simulink model "gravcomp"  (Simulink 7.5)
settings: Solver=ode3  StartTime=0.0  StopTime=inf  FixedStep=.002  RelTol=1e-3
undefined symbols (not defined in the file or in its folder): arm_home, arm_j2mt, arm_m2jp, bit, CAN_init, enc_per_rev, fdesignblkfcn, FT_init, gcbh, hand_on, MT_init, puck_I_per_Nm, rotFT2Hand, sample_time, Standard, VL1_init, VL2_init
libraries: simulink x358, xpclib x28, xpcutilitieslib x6, dspmathops x1
(part 1 of 3)
settings Model: Creator=Matt Courtney  LastModifiedBy=robotics  BufferReuse=off
settings OptimizationCC: BlockReduction=off  BooleanDataType=off  OptimizeBlockIOStorage=off  BufferReuse=off  ExpressionFolding=off  LocalBlockOutputs=off  InitFltsAndDblsToZero=on
settings DebuggingCC: StrictBusMsg=Warning
settings HardwareCC: ProdIntDivRoundTo=Zero  ProdEndianess=LittleEndian  ProdHWDeviceType=Generic->32-bit x86 compatible
settings RTWCC: SystemTargetFile=xpctarget.tlc  TemplateMakefile=xpc_default_tmf  Description=xPC Target  ProcessScript=xpctarget_make_rtw_hook  RTWCompilerOptimization=On
settings xpcTargetCC: TargetFcnLib=ansi_tfl_table_tmw.mat  TargetFunctionLibrary=ANSI_C  ERTCodeCoverageTool=None  ParMdlRefBuildCompliant=off  PortableWordSizes=off  xPCisModelTimeout=off  xPCModelTimeoutSecs=10  xPCLoadParamSetFile=off

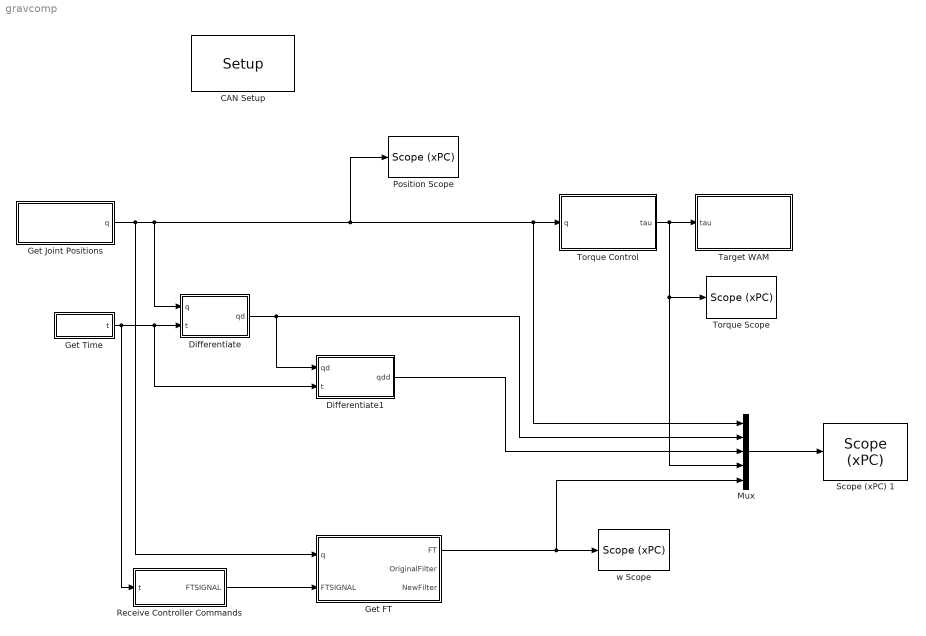
== system gravcomp ==
  "CAN Setup " : xpclib/CAN/Softing/CAN-AC2-PCI SJA 1000/Setup   board=1  can1bus=Highspeed (ISO 11898)  can1Baudrate=1 MBaud  can1UserBR=[1,1,4,3]  can2bus=Highspeed (ISO 11898)  can2Baudrate=1 MBaud  can2UserBR=[1,1,4,3]  init=[VL1_init,VL2_init,CAN_init,FT_init,MT_init]  term=[]  bus_off_out=off  bus_off_rec=Off  ioBaseAddress=-1
  Differentiate : Subsystem
  Differentiate1 : Subsystem
  Get FT : Subsystem
  Get Joint Positions : Subsystem
  Get Time : Subsystem
  Mux : Mux  Inputs=[7 7 7 7 6]
  Position Scope : xpclib/Misc./Scope (xPC)   SystemSampleTime=-1  scopeno=5  scopetype=Target  autostart=on  viewmode=Numerical  formatstr=['joint_1 %13.8f rad,joint_2 %13.8f rad,joint_3 %13.8f rad,joint_4 %13.8f rad,joint_5 %13.8f rad,joint_6 %13.8f rad,joint_7 %13.8f rad']  grid=on  ylimits=[0,0]  nosamples=1/(10*sample_time)  noprepostsamples=0  interleave=1  triggermode=FreeRun  triggersignal=1  triggerlevel=0.0  triggerslope=Either  triggerscope=1  triggersample=0  filename=data.dat  mode=Lazy  writesize=512  autorestart=off  dynamicfilemode=off  maxwritefilesize=512*1024^2
  Receive Controller Commands : Subsystem
  Scope (xPC) 1 : xpclib/Misc./Scope (xPC)   SystemSampleTime=-1  scopeno=6  scopetype=File  autostart=on  viewmode=Graphical redraw  formatstr='%15.6f'  grid=on  ylimits=[0,0]  nosamples=250  noprepostsamples=0  interleave=1  triggermode=FreeRun  triggersignal=1  triggerlevel=0.0  triggerslope=Either  triggerscope=1  triggersample=0  filename=GRAV<%%%>.dat  mode=Lazy  writesize=512  autorestart=on  dynamicfilemode=on  maxwritefilesize=512*1024^2
  Target WAM : Subsystem
  Torque Control : Subsystem
  Torque Scope : xpclib/Misc./Scope (xPC)   SystemSampleTime=-1  scopeno=1  scopetype=Target  autostart=on  viewmode=Numerical  formatstr=['joint_1 %10.5f N-m,joint_2 %10.5f N-m,joint_3 %10.5f N-m,joint_4 %10.5f N-m,joint_5 %10.5f N-m,joint_6 %10.5f N-m,joint_7 %10.5f N-m']  grid=on  ylimits=[0,0]  nosamples=1/(10*sample_time)  noprepostsamples=0  interleave=1  triggermode=FreeRun  triggersignal=1  triggerlevel=0.0  triggerslope=Either  triggerscope=1  triggersample=0  filename=data.dat  mode=Lazy  writesize=512  autorestart=off  dynamicfilemode=off  maxwritefilesize=512*1024^2
  w Scope : xpclib/Misc./Scope (xPC)   SystemSampleTime=-1  scopeno=2  scopetype=Target  autostart=on  viewmode=Numerical  formatstr=['Fx %10.5f,Fy %10.5f,Fz %10.5f,TauX %10.5f,TauY %10.5f,TauZ%10.5f']  grid=on  ylimits=[0,0]  nosamples=10  noprepostsamples=0  interleave=1  triggermode=FreeRun  triggersignal=1  triggerlevel=0.0  triggerslope=Either  triggerscope=1  triggersample=0  filename=data.dat  mode=Lazy  writesize=512  autorestart=off  dynamicfilemode=off  maxwritefilesize=512*1024^2
  wires:
  Torque Control/1(tau) -> Target WAM/1(tau), Mux/4, Torque Scope/1
  Get Joint Positions/1(q) -> Differentiate/1(q), Torque Control/1(q), Mux/1, Position Scope/1, Get FT/1(q)
  Get FT/1(FT) -> w Scope/1, Mux/5
  Mux/1 -> Scope (xPC) 1/1
  Get Time/1(t) -> Differentiate/2(t), Differentiate1/2(t), Receive Controller Commands/1(t)
  Differentiate/1(qd) -> Differentiate1/1(qd), Mux/2
  Differentiate1/1(qdd) -> Mux/3
  Receive Controller Commands/1(FTSIGNAL) -> Get FT/2(FTSIGNAL)

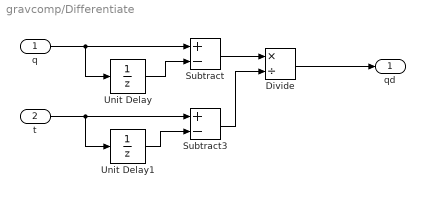
== system gravcomp/Differentiate ==
  q : Inport  OutDataType=fixdt(1, 16)  OutScaling=2^0
  t : Inport  Port=2  OutDataType=fixdt(1, 16)  OutScaling=2^0
  Divide : Product  Inputs=*/  OutDataType=fixdt(1, 16)  OutScaling=2^-10
  Subtract : Sum  Inputs=+-  OutDataType=fixdt(1, 16)  OutScaling=2^-10
  Subtract3 : Sum  Inputs=+-  OutDataType=fixdt(1, 16)  OutScaling=2^-10
  Unit Delay : UnitDelay  SampleTime=-1
  Unit Delay1 : UnitDelay  SampleTime=-1
  qd : Outport  OutDataType=fixdt(1, 16)  OutScaling=2^0
  wires:
  q/1 -> Subtract/1, Unit Delay/1
  t/1 -> Unit Delay1/1, Subtract3/1
  Unit Delay1/1 -> Subtract3/2
  Unit Delay/1 -> Subtract/2
  Subtract/1 -> Divide/1
  Divide/1 -> qd/1
  Subtract3/1 -> Divide/2

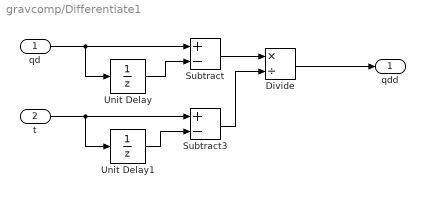
== system gravcomp/Differentiate1 ==
  qd : Inport  OutDataType=fixdt(1, 16)  OutScaling=2^0
  t : Inport  Port=2  OutDataType=fixdt(1, 16)  OutScaling=2^0
  Divide : Product  Inputs=*/  OutDataType=fixdt(1, 16)  OutScaling=2^-10
  Subtract : Sum  Inputs=+-  OutDataType=fixdt(1, 16)  OutScaling=2^-10
  Subtract3 : Sum  Inputs=+-  OutDataType=fixdt(1, 16)  OutScaling=2^-10
  Unit Delay : UnitDelay  SampleTime=-1
  Unit Delay1 : UnitDelay  SampleTime=-1
  qdd : Outport  OutDataType=fixdt(1, 16)  OutScaling=2^0
  wires:
  qd/1 -> Subtract/1, Unit Delay/1
  t/1 -> Unit Delay1/1, Subtract3/1
  Unit Delay1/1 -> Subtract3/2
  Unit Delay/1 -> Subtract/2
  Subtract/1 -> Divide/1
  Divide/1 -> qdd/1
  Subtract3/1 -> Divide/2

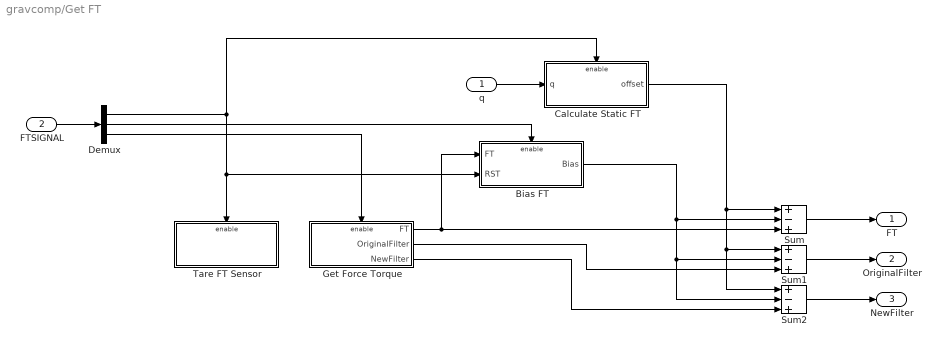
== system gravcomp/Get FT ==
  q : Inport  OutDataType=fixdt(1, 16)  OutScaling=2^0
  FTSIGNAL : Inport  Port=2  OutDataType=fixdt(1, 16)  OutScaling=2^0
  Bias FT : Subsystem  TreatAsAtomicUnit=on
  Calculate Static FT : Subsystem  TreatAsAtomicUnit=on
  Demux : Demux  Outputs=3
  Get Force Torque : Subsystem
  Sum : Sum  Inputs=+-+  OutDataType=fixdt(1, 16)  OutScaling=2^0
  Sum1 : Sum  Inputs=+-+  OutDataType=fixdt(1, 16)  OutScaling=2^0
  Sum2 : Sum  Inputs=+-+  OutDataType=fixdt(1, 16)  OutScaling=2^0
  Tare FT Sensor : Subsystem  TreatAsAtomicUnit=on
  FT : Outport  OutDataType=fixdt(1, 16)  OutScaling=2^0
  OriginalFilter : Outport  Port=2  OutDataType=fixdt(1, 16)  OutScaling=2^0
  NewFilter : Outport  Port=3  OutDataType=fixdt(1, 16)  OutScaling=2^0
  wires:
  FTSIGNAL/1 -> Demux/1
  Demux/1 -> Tare FT Sensor/Enable, Bias FT/2(RST), Calculate Static FT/Enable
  Demux/3 -> Get Force Torque/Enable
  Demux/2 -> Bias FT/Enable
  Get Force Torque/1(FT) -> Bias FT/1(FT), Sum/3
  Sum/1 -> FT/1
  Bias FT/1(Bias) -> Sum/2, Sum2/2, Sum1/2
  Get Force Torque/2(OriginalFilter) -> Sum1/3
  Get Force Torque/3(NewFilter) -> Sum2/3
  Sum2/1 -> NewFilter/1
  Sum1/1 -> OriginalFilter/1
  q/1 -> Calculate Static FT/1(q)
  Calculate Static FT/1(offset) -> Sum/1, Sum1/1, Sum2/1

== system gravcomp/Get Joint Positions ==
  DocBlock : simulink/Model-Wide Utilities/DocBlock  SystemSampleTime=-1  DocumentType=Text
  Motor Counts to Joint Radians1 : Subsystem
  Recieve and Unpack  Motor Positions1 : Subsystem
  Send: GetPosition : Subsystem
  q : Outport  OutDataType=sfix(16)  OutScaling=2^0
  wires:
  Motor Counts to Joint Radians1/1(qJ) -> q/1
  Recieve and Unpack  Motor Positions1/1(qM) -> Motor Counts to Joint Radians1/1(qM)

== system gravcomp/Get Time ==
  Clock Frequency : Constant  Value=1.193e6  OutDataType=fixdt(1, 16)  OutScaling=2^0
  Divide1 : Product  Inputs=*/  OutDataType=fixdt(1, 16)  OutScaling=2^-10
  "xPC Target  Time " : xpclib/Misc./xPC Target  Time   ts=sample_time
  t : Outport  OutDataType=fixdt(1, 16)  OutScaling=2^0
  wires:
  "xPC Target  Time "/1 -> Divide1/1
  Clock Frequency/1 -> Divide1/2
  Divide1/1 -> t/1

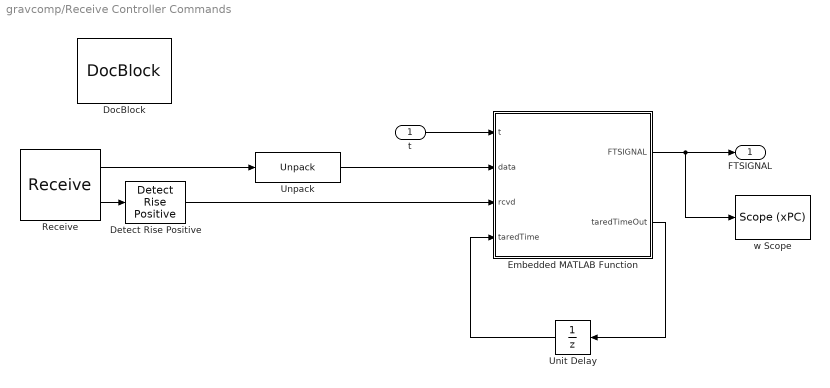
== system gravcomp/Receive Controller Commands ==
  t : Inport  OutDataType=fixdt(1, 16)  OutScaling=2^0
  Detect Rise Positive : simulink/Logic and Bit Operations/Detect Rise Positive  SystemSampleTime=-1  vinit=0
  DocBlock : simulink/Model-Wide Utilities/DocBlock  SystemSampleTime=-1  DocumentType=Text
  Embedded MATLAB Function : Stateflow chart  TreatAsAtomicUnit=on
  Receive : xpclib/UDP/Receive  ipAddress=192.168.1.11  ipPort=6666  width=9  vblLen=off  sampletime=sample_time
  Unit Delay : UnitDelay  SampleTime=-1
  Unpack : xpclib/UDP/Unpack  dimensions={[9,1]}  datatypes={'uint8'}  byteAlign=1
  w Scope : xpclib/Misc./Scope (xPC)   SystemSampleTime=-1  scopeno=3  scopetype=Target  autostart=on  viewmode=Numerical  formatstr=['%10.5f']  grid=on  ylimits=[0,0]  nosamples=10  noprepostsamples=0  interleave=1  triggermode=FreeRun  triggersignal=1  triggerlevel=0.0  triggerslope=Either  triggerscope=1  triggersample=0  filename=data.dat  mode=Lazy  writesize=512  autorestart=off  dynamicfilemode=off  maxwritefilesize=512*1024^2
  FTSIGNAL : Outport  OutDataType=fixdt(1, 16)  OutScaling=2^0
  wires:
  Receive/1 -> Unpack/1
  Receive/2 -> Detect Rise Positive/1
  Detect Rise Positive/1 -> Embedded MATLAB Function/3(rcvd)
  Unpack/1 -> Embedded MATLAB Function/2(data)
  t/1 -> Embedded MATLAB Function/1(t)
  Embedded MATLAB Function/2(taredTimeOut) -> Unit Delay/1
  Unit Delay/1 -> Embedded MATLAB Function/4(taredTime)
  Embedded MATLAB Function/1(FTSIGNAL) -> FTSIGNAL/1, w Scope/1

== system gravcomp/Target WAM ==
  tau : Inport  OutDataType=sfix(16)  OutScaling=2^0
  Check WAM MODE : Subsystem
  DocBlock : simulink/Model-Wide Utilities/DocBlock  SystemSampleTime=-1  DocumentType=Text
      content=|
      | This block does all of the communication with the WAM over the CAN card.
      | First we check the WAM mode to see if it in is Shift-Idle or Shift-Active
      | mode. It is necessary to pass this as output, so that PID knows whether it
      | should be integrating on the error or not. If we are in Shift-Idle mode,
      | we send zero torques. Also in this block, we convert joint torque to motor
      | current using the transformations in the documentation. Then we pack the
      | torque packets into a CAN message and send it.
      |
      | To receive joint positions we also send a CAN message which will respond
      | back with the appropriate information. Once we receive the joint positions,
      | we need to differentiate it to get joint velocities (since the WAM does not
      | have tachometers). Finally, passing it through a moving average of the last
      | n readings removes some of the noise and gives us a smoother velocity
      | signal.
  Joint Torque to Motor Current1 : Subsystem
  Pack and Send Torque Packets : Subsystem
  Switch : Switch  Threshold=2  OutDataType=sfix(16)  OutScaling=2^0
  Zero Torques : Constant  Value=[ 0 0 0 0 0 0 0]'  OutDataTypeMode=int16  OutDataType=sfix(16)  OutScaling=2^0  OutDataTypeStr=int16
  wires:
  Joint Torque to Motor Current1/1(iM) -> Pack and Send Torque Packets/1(Current)
  Switch/1 -> Joint Torque to Motor Current1/1(tauJ)
  tau/1 -> Switch/1
  Zero Torques/1 -> Switch/3
  Check WAM MODE/1(MODE) -> Switch/2

== system gravcomp/Torque Control ==
  q : Inport  OutDataType=sfix(16)  OutScaling=2^0
  Constant1 : Constant  Value=hand_on  OutDataType=fixdt(1, 16)  OutScaling=2^0
  Gravity Comp : Stateflow chart  TreatAsAtomicUnit=on
  tau : Outport  OutDataType=sfix(16)  OutScaling=2^0
  wires:
  q/1 -> Gravity Comp/2(q)
  Gravity Comp/1(tau) -> tau/1
  Constant1/1 -> Gravity Comp/1(hand_on)

== system gravcomp/Get FT/Bias FT ==
  FT : Inport  OutDataType=fixdt(1, 16)  OutScaling=2^0
  RST : Inport  Port=2  OutDataType=fixdt(1, 16)  OutScaling=2^0
  Enable : EnablePort  StatesWhenEnabling=reset
  Constant : Constant  Value=500  OutDataType=fixdt(1, 16)  OutScaling=2^0
  Cumulative Sum : dspmathops/Cumulative Sum  DialogController=dspDDGCreate  DialogControllerArgs=DataTag0  dim=Channels (running sum)  reset_popup=Non-zero sample  outputDataTypeStr=Inherit: Same as accumulator  outputLastDataTypeStr=Inherit: Same as accumulator  outputMin=[]  outputMax=[]  roundingMode=Floor  overflowMode=off
  Product : Product  Inputs=*/  OutDataType=fixdt(1, 16)  OutScaling=2^0  RndMeth=Zero
  Bias : Outport  OutDataType=fixdt(1, 16)  OutScaling=2^0
  wires:
  FT/1 -> Cumulative Sum/1
  RST/1 -> Cumulative Sum/2
  Constant/1 -> Product/2
  Cumulative Sum/1 -> Product/1
  Product/1 -> Bias/1

== system gravcomp/Get FT/Calculate Static FT ==
  q : Inport  OutDataType=fixdt(1, 16)  OutScaling=2^0
  Enable : EnablePort  StatesWhenEnabling=reset
  Constant1 : Constant  Value=hand_on  OutDataType=fixdt(1, 16)  OutScaling=2^0
  StaticFT : Stateflow chart  TreatAsAtomicUnit=on
  offset : Outport  OutDataType=fixdt(1, 16)  OutScaling=2^0
  wires:
  q/1 -> StaticFT/1(q)
  StaticFT/1(FTExp) -> offset/1
  Constant1/1 -> StaticFT/2(hand_on)

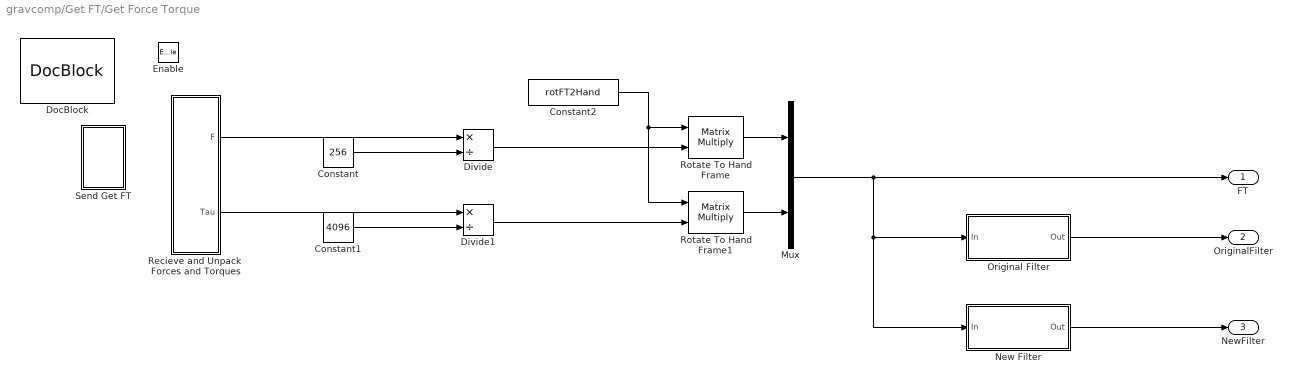
== system gravcomp/Get FT/Get Force Torque ==
  Enable : EnablePort
  Constant : Constant  Value=256  OutDataType=fixdt(1, 16)  OutScaling=2^0
  Constant1 : Constant  Value=4096  OutDataType=fixdt(1, 16)  OutScaling=2^0
  Constant2 : Constant  Value=rotFT2Hand  OutDataType=fixdt(1, 16)  OutScaling=2^0
  Divide : Product  Inputs=*/  OutDataType=fixdt(1, 16)  OutScaling=2^-10
  Divide1 : Product  Inputs=*/  OutDataType=fixdt(1, 16)  OutScaling=2^-10
  DocBlock : simulink/Model-Wide Utilities/DocBlock  SystemSampleTime=-1  DocumentType=Text
  Mux : Mux  Inputs=2
  New Filter : Subsystem  DialogController=fdesignblkfcn  DialogControllerArgs=DataTag3  InitFcn=fdesignblkfcn(gcbh, {'InitFcn'});
      settings: CopyFcn=fdesignblkfcn(gcbh, {'CopyFcn'});
      mask Type: Lowpass Filter
      mask Description: Design a lowpass filter
      mask Help: helpview(mapfilelocation('dspblks'), 'dsplowpassfilter')
      mask Display: disp('Lowpass')
  Original Filter : Subsystem  DialogController=fdesignblkfcn  DialogControllerArgs=DataTag6  InitFcn=fdesignblkfcn(gcbh, {'InitFcn'});
      settings: CopyFcn=fdesignblkfcn(gcbh, {'CopyFcn'});
      mask Type: Lowpass Filter
      mask Description: Design a lowpass filter
      mask Help: helpview(mapfilelocation('dspblks'), 'dsplowpassfilter')
      mask Display: disp('Lowpass')
  Recieve and Unpack  Forces and Torques : Subsystem
  Rotate To Hand Frame : Product  Multiplication=Matrix(*)  OutDataType=sfix(16)  OutScaling=2^0
  Rotate To Hand Frame1 : Product  Multiplication=Matrix(*)  OutDataType=sfix(16)  OutScaling=2^0
  Send Get FT : Subsystem
  FT : Outport  OutDataType=fixdt(1, 16)  OutScaling=2^0
  OriginalFilter : Outport  Port=2  OutDataType=fixdt(1, 16)  OutScaling=2^0
  NewFilter : Outport  Port=3  OutDataType=fixdt(1, 16)  OutScaling=2^0
  wires:
  Constant/1 -> Divide/2
  Constant1/1 -> Divide1/2
  Rotate To Hand Frame/1 -> Mux/1
  Rotate To Hand Frame1/1 -> Mux/2
  Constant2/1 -> Rotate To Hand Frame1/1, Rotate To Hand Frame/1
  Recieve and Unpack  Forces and Torques/2(Tau) -> Divide1/1
  Recieve and Unpack  Forces and Torques/1(F) -> Divide/1
  Divide/1 -> Rotate To Hand Frame/2
  Divide1/1 -> Rotate To Hand Frame1/2
  Mux/1 -> FT/1, New Filter/1(In), Original Filter/1(In)
  Original Filter/1(Out) -> OriginalFilter/1
  New Filter/1(Out) -> NewFilter/1

== system gravcomp/Get FT/Tare FT Sensor ==
  Enable : EnablePort
  ANY VALUE : Constant  Value=[0]  OutDataTypeMode=uint8  OutDataType=sfix(16)  OutScaling=2^0  OutDataTypeStr=uint8
  Bit Packing : xpcutilitieslib/Bit Packing   MaskBitPatterns={[0:7] [8:39] [40:55]}  MaskPackDataType=double  MaskPackDataSize=[1]
  Data Type Conversion1 : DataTypeConversion  OutMin=[-8191]  OutMax=[8191]  OutDataTypeMode=int32  OutDataType=int14  OutDataTypeStr=int32  RndMeth=Zero
  Send To FT : xpclib/CAN/Softing/CAN-AC2-PCI SJA 1000/Send   board=1  canPort=CAN 1  range=Standard (11-bit)  ids=bin2dec('00000001000')  sizes=[8]  output=off  ts=sample_time  ididx=[0]
  TARE FT : Constant  Value=[182]  OutDataTypeMode=uint8  OutDataType=sfix(16)  OutScaling=2^0  OutDataTypeStr=uint8
  wires:
  TARE FT/1 -> Bit Packing/1
  Bit Packing/1 -> Send To FT/1
  ANY VALUE/1 -> Data Type Conversion1/1
  Data Type Conversion1/1 -> Bit Packing/2, Bit Packing/3

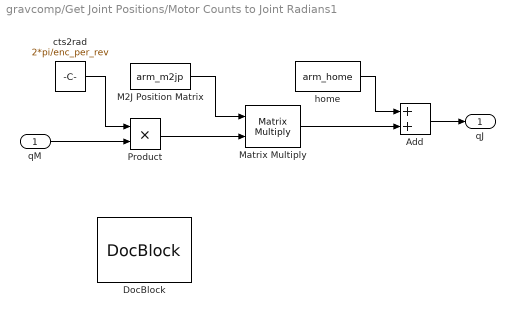
== system gravcomp/Get Joint Positions/Motor Counts to Joint Radians1 ==
  qM : Inport  OutDataType=fixdt(1, 16)  OutScaling=2^0
  Add : Sum  OutDataType=fixdt(1, 16)  OutScaling=2^-10
  DocBlock : simulink/Model-Wide Utilities/DocBlock  SystemSampleTime=-1  DocumentType=Text
      content=|
      | Here we do the simple conversion from motor position to joint position,
      | then convert encoder counts to joint radians, then account for the offset
      | in the home position to finally output the joint position in radians. The
      | M2J position matrix can be found in the documentation. Joint 4 has a -18 as
      | opposed to +18 because the motor was reversed at one point during a repair.
      | I believe newer models of the WAM adhere to this -18.
  M2J Position Matrix : Constant  Value=arm_m2jp  OutDataType=fixdt(1, 16)  OutScaling=2^0
  Matrix Multiply : Product  Multiplication=Matrix(*)  OutDataType=sfix(16)  OutScaling=2^0
  Product : Product  OutMin=[-8192]  OutMax=[8191]  OutDataType=fixdt(1, 16)  OutScaling=2^0  RndMeth=Zero
  cts2rad : Constant  Value=2*pi/enc_per_rev  OutDataType=fixdt(1, 16)  OutScaling=2^0
  home : Constant  Value=arm_home  OutDataType=fixdt(1, 16)  OutScaling=2^0
  qJ : Outport  OutDataType=fixdt(1, 16)  OutScaling=2^0
  wires:
  qM/1 -> Product/2
  Add/1 -> qJ/1
  Matrix Multiply/1 -> Add/2
  home/1 -> Add/1
  cts2rad/1 -> Product/1
  M2J Position Matrix/1 -> Matrix Multiply/1
  Product/1 -> Matrix Multiply/2

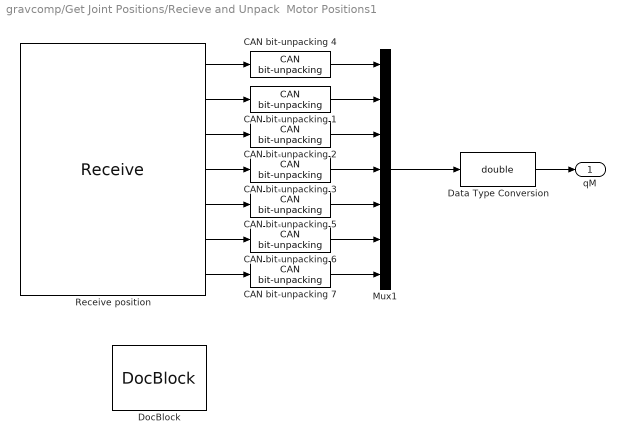
== system gravcomp/Get Joint Positions/Recieve and Unpack  Motor Positions1 ==
  CAN bit-unpacking {1..7} (7 alike) : xpclib/CAN/Utilities/CAN bit-unpacking   bitpatterns={ [16:23, 8:15, 0:5,-1, -1] }  dtypes={ 'int32'}
  Data Type Conversion : DataTypeConversion  OutDataTypeMode=double  OutDataType=sfix(16)  OutScaling=2^0  OutDataTypeStr=double
  DocBlock : simulink/Model-Wide Utilities/DocBlock  SystemSampleTime=-1  DocumentType=Text
  Mux1 : Mux  Inputs=7
  "Receive position " : xpclib/CAN/Softing/CAN-AC2-PCI SJA 1000/Receive   board=1  canPort=CAN 1  range=Standard (11-bit)  ids=[bin2dec('10000100011'),bin2dec('10001000011'),bin2dec('10001100011'),bin2dec('10010000011'),bin2dec('10010100011'),bin2dec('10011000011'),bin2dec('10011100011')]  lengths=0  output=Data  inten=on  ts=sample_time  ididx=[0,1,2,3,5,6,7]
  qM : Outport
  wires:
  Mux1/1 -> Data Type Conversion/1
  "Receive position "/1 -> CAN bit-unpacking 4/1
  "Receive position "/2 -> CAN bit-unpacking 1/1
  "Receive position "/3 -> CAN bit-unpacking 2/1
  "Receive position "/4 -> CAN bit-unpacking 3/1
  CAN bit-unpacking 4/1 -> Mux1/1
  CAN bit-unpacking 1/1 -> Mux1/2
  CAN bit-unpacking 2/1 -> Mux1/3
  CAN bit-unpacking 3/1 -> Mux1/4
  Data Type Conversion/1 -> qM/1
  "Receive position "/5 -> CAN bit-unpacking 5/1
  "Receive position "/6 -> CAN bit-unpacking 6/1
  "Receive position "/7 -> CAN bit-unpacking 7/1
  CAN bit-unpacking 5/1 -> Mux1/5
  CAN bit-unpacking 6/1 -> Mux1/6
  CAN bit-unpacking 7/1 -> Mux1/7

== system gravcomp/Get Joint Positions/Send: GetPosition ==
  Bit Packing : xpcutilitieslib/Bit Packing   MaskBitPatterns={[0:7]}  MaskPackDataType=double  MaskPackDataSize=[1]
  DocBlock : simulink/Model-Wide Utilities/DocBlock  SystemSampleTime=-1  DocumentType=Text
  Send to all motors : xpclib/CAN/Softing/CAN-AC2-PCI SJA 1000/Send   board=1  canPort=CAN 1  range=Standard (11-bit)  ids=1024  sizes=[1]  output=off  ts=sample_time  ididx=[2]
  get position : Constant  Value=[48]  OutDataTypeMode=int8  OutDataType=sfix(16)  OutScaling=2^0  OutDataTypeStr=int8
  wires:
  Bit Packing/1 -> Send to all motors/1
  get position/1 -> Bit Packing/1

== system gravcomp/Target WAM/Check WAM MODE ==
  note: Send to lower arm
  "Bit Packing " : xpcutilitieslib/Bit Packing   MaskBitPatterns={[0:7]}  MaskPackDataType=double  MaskPackDataSize=[1]
  Bit Unpacking : xpclib/CAN/Utilities/CAN bit-unpacking   bitpatterns={[16:31]}  dtypes={ 'int16'}
  DocBlock : simulink/Model-Wide Utilities/DocBlock  SystemSampleTime=-1  DocumentType=Text
      content=|
      | Here we send an 8 to the lower arm. Property 8 is the MODE and the
      | 1028 (1 00000 00100) means to "set a lower arm property". Finally we
      | receive the mode property from CAN ID 1158, then do some bit unpacking.
      | All of this is well documentated in the "CAN Communication Spec" of the
      | Barrett documentation.
  Receive lower arm property : xpclib/CAN/Softing/CAN-AC2-PCI SJA 1000/Receive   board=1  canPort=CAN 1  range=Standard (11-bit)  ids=[bin2dec('10010000110')]  lengths=0  output=Data  inten=on  ts=sample_time  ididx=[4]
  Send to all motors 1 : xpclib/CAN/Softing/CAN-AC2-PCI SJA 1000/Send   board=1  canPort=CAN 1  range=Standard (11-bit)  ids=[1028]  sizes=[1]  output=off  ts=sample_time  ididx=[5]
  get MODE : Constant  Value=[8]  OutDataTypeMode=uint8  OutDataType=sfix(16)  OutScaling=2^0  OutDataTypeStr=uint8
  MODE : Outport  OutDataType=sfix(16)  OutScaling=2^0
  wires:
  "Bit Packing "/1 -> Send to all motors 1/1
  Receive lower arm property/1 -> Bit Unpacking/1
  get MODE/1 -> "Bit Packing "/1
  Bit Unpacking/1 -> MODE/1

== system gravcomp/Target WAM/Joint Torque to Motor Current1 ==
  tauJ : Inport  OutDataType=fixdt(1, 16)  OutScaling=2^0
  DocBlock : simulink/Model-Wide Utilities/DocBlock  SystemSampleTime=-1  DocumentType=Text
  J2M Torque Matrix : Constant  Value=arm_j2mt  OutDataType=fixdt(1, 16)  OutScaling=2^0
  Matrix Multiply : Product  Multiplication=Matrix(*)  OutDataType=sfix(16)  OutScaling=2^0
  Product : Product  OutDataType=fixdt(1, 16)  OutScaling=2^0  RndMeth=Zero
  puckIperNm : Constant  Value=puck_I_per_Nm  OutDataType=fixdt(1, 16)  OutScaling=2^0
  iM : Outport  OutDataType=fixdt(1, 16)  OutScaling=2^0
  wires:
  J2M Torque Matrix/1 -> Matrix Multiply/1
  Matrix Multiply/1 -> Product/2
  puckIperNm/1 -> Product/1
  Product/1 -> iM/1
  tauJ/1 -> Matrix Multiply/2

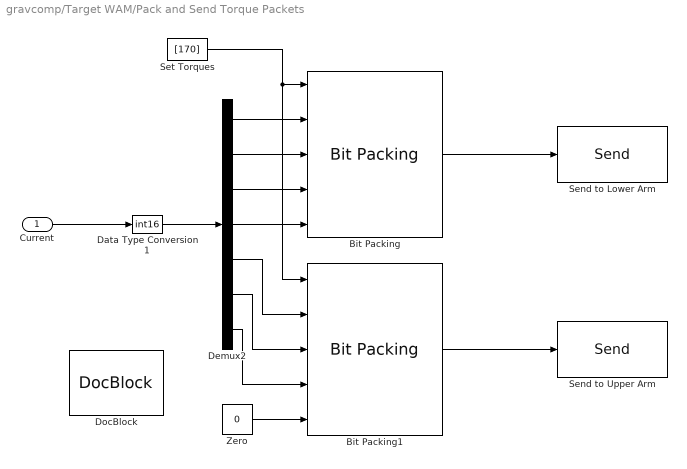
== system gravcomp/Target WAM/Pack and Send Torque Packets ==
  Current : Inport
  Bit Packing : xpcutilitieslib/Bit Packing   MaskBitPatterns={[0:7] [18:23 8:15] [36:39 24:31 16:17] [54:55 40:47 32:35] [56:63 48:53]}  MaskPackDataType=double  MaskPackDataSize=[1]
  Bit Packing1 : xpcutilitieslib/Bit Packing   MaskBitPatterns={[0:7] [18:23 8:15] [36:39 24:31 16:17] [54:55 40:47 32:35] [56:63 48:53]}  MaskPackDataType=double  MaskPackDataSize=[1]
  Data Type Conversion1 : DataTypeConversion  OutMin=[-8191]  OutMax=[8191]  OutDataTypeMode=int16  OutDataType=int14  OutDataTypeStr=int16  RndMeth=Zero
  Demux2 : Demux  Outputs=7
  DocBlock : simulink/Model-Wide Utilities/DocBlock  SystemSampleTime=-1  DocumentType=Text
  Send to Lower Arm : xpclib/CAN/Softing/CAN-AC2-PCI SJA 1000/Send   board=1  canPort=CAN 1  range=Standard (11-bit)  ids=bin2dec('10000000001')  sizes=[8]  output=off  ts=sample_time  ididx=[3]
  Send to Upper Arm : xpclib/CAN/Softing/CAN-AC2-PCI SJA 1000/Send   board=1  canPort=CAN 1  range=Standard (11-bit)  ids=bin2dec('10000000010')  sizes=[8]  output=off  ts=sample_time  ididx=[4]
  "Set Torques " : Constant  Value=[170]  OutDataTypeMode=uint8  OutDataType=sfix(16)  OutScaling=2^0  OutDataTypeStr=uint8
  Zero : Constant  Value=0  OutDataTypeMode=int16  OutDataType=fixdt(1, 16)  OutScaling=2^0  OutDataTypeStr=int16
  wires:
  "Set Torques "/1 -> Bit Packing/1, Bit Packing1/1
  Bit Packing/1 -> Send to Lower Arm/1
  Demux2/1 -> Bit Packing/2
  Demux2/2 -> Bit Packing/3
  Demux2/3 -> Bit Packing/4
  Demux2/4 -> Bit Packing/5
  Current/1 -> Data Type Conversion1/1
  Data Type Conversion1/1 -> Demux2/1
  Bit Packing1/1 -> Send to Upper Arm/1
  Demux2/5 -> Bit Packing1/2
  Demux2/6 -> Bit Packing1/3
  Demux2/7 -> Bit Packing1/4
  Zero/1 -> Bit Packing1/5

== system gravcomp/Get FT/Get Force Torque/New Filter ==
  In : Inport  OutDataType=sfix(16)  OutScaling=2^0
  Generated Filter Block : Subsystem  Tag=FilterWizardSubSystem
      settings: ErrorFcn=dspFilterRealizedInBasicElemsAlgLoopErrFcnCallback
  Out : Outport  OutDataType=sfix(16)  OutScaling=2^0
  wires:
  In/1 -> Generated Filter Block/1(Input)
  Generated Filter Block/1(Output) -> Out/1

== system gravcomp/Get FT/Get Force Torque/Original Filter ==
  In : Inport  OutDataType=sfix(16)  OutScaling=2^0
  Generated Filter Block : Subsystem  Tag=FilterWizardSubSystem
      settings: ErrorFcn=dspFilterRealizedInBasicElemsAlgLoopErrFcnCallback
  Out : Outport  OutDataType=sfix(16)  OutScaling=2^0
  wires:
  In/1 -> Generated Filter Block/1(Input)
  Generated Filter Block/1(Output) -> Out/1

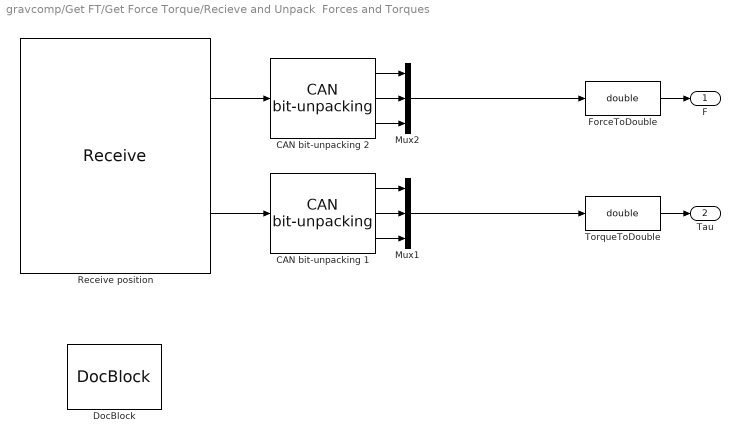
== system gravcomp/Get FT/Get Force Torque/Recieve and Unpack  Forces and Torques ==
  CAN bit-unpacking 1 : xpclib/CAN/Utilities/CAN bit-unpacking   bitpatterns={[0:15],[16:31],[32:47]}  dtypes={'int32','int32','int32'}
  CAN bit-unpacking 2 : xpclib/CAN/Utilities/CAN bit-unpacking   bitpatterns={[0:15],[16:31],[32:47]}  dtypes={'int32','int32','int32'}
  DocBlock : simulink/Model-Wide Utilities/DocBlock  SystemSampleTime=-1  DocumentType=Text
  ForceToDouble : DataTypeConversion  OutDataTypeMode=double  OutDataType=sfix(16)  OutScaling=2^0  OutDataTypeStr=double
  Mux1 : Mux  Inputs=3
  Mux2 : Mux  Inputs=3
  "Receive position " : xpclib/CAN/Softing/CAN-AC2-PCI SJA 1000/Receive   board=1  canPort=CAN 1  range=Standard (11-bit)  ids=[bin2dec('10100001010'),bin2dec('10100001011')]  lengths=0  output=Data  inten=on  ts=sample_time  ididx=[8,9]
  TorqueToDouble : DataTypeConversion  OutDataTypeMode=double  OutDataType=sfix(16)  OutScaling=2^0  OutDataTypeStr=double
  F : Outport
  Tau : Outport  Port=2
  wires:
  "Receive position "/1 -> CAN bit-unpacking 2/1
  "Receive position "/2 -> CAN bit-unpacking 1/1
  Mux1/1 -> TorqueToDouble/1
  CAN bit-unpacking 1/1 -> Mux1/1
  CAN bit-unpacking 1/2 -> Mux1/2
  CAN bit-unpacking 1/3 -> Mux1/3
  TorqueToDouble/1 -> Tau/1
  ForceToDouble/1 -> F/1
  CAN bit-unpacking 2/1 -> Mux2/1
  CAN bit-unpacking 2/2 -> Mux2/2
  CAN bit-unpacking 2/3 -> Mux2/3
  Mux2/1 -> ForceToDouble/1

== system gravcomp/Get FT/Get Force Torque/Send Get FT ==
  Bit Packing : xpcutilitieslib/Bit Packing   MaskBitPatterns={[0:7]}  MaskPackDataType=double  MaskPackDataSize=[1]
  Send to FTsensor : xpclib/CAN/Softing/CAN-AC2-PCI SJA 1000/Send   board=1  canPort=CAN 1  range=Standard (11-bit)  ids=bin2dec('00000001000')  sizes=[1]  output=off  ts=sample_time  ididx=[0]
  get FT : Constant  Value=[54]  OutDataTypeMode=int8  OutDataType=sfix(16)  OutScaling=2^0  OutDataTypeStr=int8
  wires:
  get FT/1 -> Bit Packing/1
  Bit Packing/1 -> Send to FTsensor/1
